simulink model "new_model_like_me"  (R2023a)
settings: Solver=FixedStepDiscrete  StartTime=0.0  StopTime=5  FixedStep=Ts  RelTol=1e-3  EnableMultiTasking=on
PreLoadFcn:
  | parameters_for_model_inn;
StopFcn:
  | ee_addSimlogTimeStamp(bdroot)
values from neighbouring files (symbols this model uses):
  deg = 10    [parameters_for_model_inn.m]
  Jm = 0.001368    [parameters_for_model_inn.m]
  Kaw_omega = 1    [parameters_for_model_inn.m]
  Ki_id = 3    [parameters_for_model_inn.m]
  Ki_iq = 20    [parameters_for_model_inn.m]
  Ki_omega = 2.2    [parameters_for_model_inn.m]
  Kp_id = 0.01    [parameters_for_model_inn.m]
  Kp_iq = 1.8    [parameters_for_model_inn.m]
  Kp_omega = 0.6    [parameters_for_model_inn.m]
  Kp_pos = 0.8    [parameters_for_model_inn.m]
  Ld = 0.00595    [parameters_for_model_inn.m]
  LimA2down = -80    [parameters_for_model_inn.m]
  LimA2up = 64    [parameters_for_model_inn.m]
  Lq = 0.00595    [parameters_for_model_inn.m]
  p = 4    [parameters_for_model_inn.m]
  psim = 0.180694733685904    (= 0.180694733686)    [parameters_for_model_inn.m]
  Red = 34.68    [parameters_for_model_inn.m]
  Tid_start = Tiq_stop + 0.02    (= 0.1)    [parameters_for_model_inn.m]
  Tid_stop = Tid_start + 0.04    (= 0.14)    [parameters_for_model_inn.m]
  Tiq_start = 0.02    [parameters_for_model_inn.m]
  Tiq_stop = Tiq_start + 0.06    (= 0.08)    [parameters_for_model_inn.m]
  Tomega_start = Tid_stop + 0.02    (= 0.16)    [parameters_for_model_inn.m]
  Tomega_stop = Tomega_start + 0.06    (= 0.22)    [parameters_for_model_inn.m]
  Tpos_start = Tomega_stop + 0.02    (= 0.24)    [parameters_for_model_inn.m]
  Tpos_stop = Tpos_start + 0.06    (= 0.3)    [parameters_for_model_inn.m]
  Ts = 5e-5    (= 5e-05)    [parameters_for_model_inn.m]
  Tsi = Ts * 20    (= 0.001)    [parameters_for_model_inn.m]
  Tso = Ts * 200    (= 0.01)    [parameters_for_model_inn.m]
  V1 = 250    [parameters_for_model_inn.m]
  Vnom = 300    [parameters_for_model_inn.m]
  Wmax = 7000    [parameters_for_model_inn.m]
  Wnom = 1800    [parameters_for_model_inn.m]
undefined symbols (not defined in the file or in its folder): DiscIntNeverNeededParam, Kd_pos, Ki_pos, Kn_pos, Tpos, X, Y, Z
libraries: nesl_utility x18, fl_lib x10, sm_lib x8, slctrlblks x6, ee_lib x5, eeTransforms x3, dspfdesign x3, eePmsmCurrentController x2, simulink x2, slpidlib x2, robotmaniplib x2, batteryecm_lib x1
(part 2 of 2)

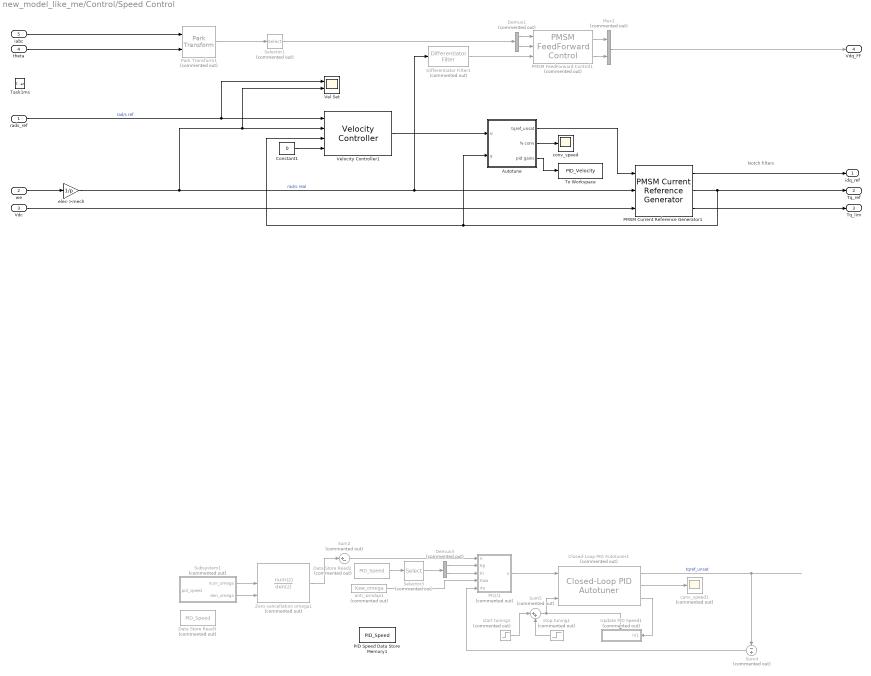
== system new_model_like_me/Control/Speed Control ==
  note: Notch filters
  rads_ref : Inport
  we : Inport  Port=2
  Vdc : Inport  Port=3
  theta : Inport  Port=4
  iabc : Inport  Port=5
  Task1ms : TriggerPort  TriggerType=function-call  VariantControl=Variant  PortDimensions=1
  Autotune : Subsystem
  Closed-Loop PID Autotuner1 : slctrlblks/Closed-Loop PID Autotuner  Commented=on  PIDType=PI  PIDForm=Parallel  TimeDomain=discrete-time  DiscreteTs=-1  TuningTs=0.2  UseTuningTs=off  IntegratorFormula=Forward Euler  FilterFormula=Forward Euler  ContinuousTs=0.02  Bandwidth=Wnom*(2*pi/60)  UseExternalWC=off  TargetPM=60  UseExternalPM=off  UseExternalAchievedPM=off  ExperimentMode=Superposition  PlantType=Stable  PlantSign=Positive  AmpSine=0.3  UseExternalAmpSine=off  UseExternalFRD=off  UseExternalU0=off  UseCompanion=off  NotDeployTuningModule=off  UsePLCCoder=off  OutputMode=control action + perturbation  BlockDataType=double  UseConnectedPID=on  blockpath=[]  tunedP=0  tunedI=0  tunedD=0  tunedN=100  tunedPM=0  EstimationWindowSize=3  UseExternalTuningParams=off  SingleMultiRateVariant=SingleSamplingRate  NumEstimationPeriods=4  NumSettlingPeriods=2  ExperimentModeVariant=VariantSuperimposed  OutputChoice=VariantCandD
  Constant1 : Constant  Value=0  SampleTime=-1
  Data Store Read2 : DataStoreRead  Commented=on  DataStoreName=PID_Speed  IndexOptions=Index vector (dialog)  Indices=1  OutputSizes=1
  Data Store Read3 : DataStoreRead  Commented=on  DataStoreName=PID_Speed  IndexOptions=Index vector (dialog)  Indices=1  OutputSizes=1
  Demux1 : Demux  Commented=on  Outputs=2
  Demux3 : Demux  Commented=on  Outputs=2
  Differentiator Filter1 : dspfdesign/Differentiator Filter  Commented=on  DesignForMinimumOrder=on  FilterOrder=31  PassbandRipple=0.1  ScaleCoefficients=off  SimulateUsing=Interpreted execution  roundingMode=Floor  coeffsDataTypeStr=fixdt(1,16)
  Mux1 : Mux  Commented=on  Inputs=2
  PI(z)1 : Subsystem  Commented=on
  PID Speed Data Store Memory1 : DataStoreMemory  DataStoreName=PID_Speed  InitialValue=[Kp_omega Ki_omega 0 Kaw_omega]  ShowAdditionalParam=off
  PMSM Current Reference Generator1 : eePmsmCurrentReferenceGen/PMSM Current Reference Generator  Vnom=Vnom  Pmax=Pmax  Tmax=Tmax  Ts=-1  RefType=Zero d-axis control  rpmVec=RPM_VECT  TqVec=TQ_VECT  VdcVec=VDC_VECT  PWMMode=SVM: space vector modulation  ModFactor=1  idMatrix=ID_MAP  iqMatrix=IQ_MAP  p=p  psim=psim  Ld=Ld  Lq=Lq  Rs=Rs  RefExpEnable=1
  PMSM FeedForward Control1 : mcbpmsmnonlinearlib/PMSM FeedForward Control  Commented=on  polePairs=p  nonLinearityChoice=Linear model with lumped parameters  Ld=Ld  Lq=Lq  FluxPM=psim  idVec=[-40, -20, 0, 20]  iqVec=[-40, -20, 0, 20, 40]  LdTable=0.2e-3 * ones(4, 5)  LqTable=0.2e-3 * ones(4, 5)  FluxPMTable=6.4e-3 * ones(4, 5)  FluxDTable=[-1.6,-1.6,-1.6,-1.6,-1.6;2.4,2.4,2.4,2.4,2.4;6.4,6.4,6.4,6.4,6.4;10.4,10.4,10.4,10.4,10.4]*1e-3  FluxQTable=[-8,-4,0,4,8;-8,-4,0,4,8;-8,-4,0,4,8;-8,-4,0,4,8]*1e-3  Vsat_input_select=Specify via dialog  v_sat=Vnom/sqrt(3)  Units=Per-Unit (PU)  V_base=Vnom/sqrt(3)  I_base=Imax  N_base=Wmax  scaledTables=on
      settings: LibrarySourceBlock=mcblib/Controls/Control Reference/PMSM FeedForward Control
  Park Transform1 : eeTransforms/Park Transform  Commented=on  AxisAlignment=Q-axis  PowerInvariant=off
      settings: LibrarySourceBlock=|
      | ee_sl_lib/Mathematical
      | Transforms/Park Transform
  Selector1 : Selector  Commented=on  InputPortWidth=3  IndexOptions=Index vector (dialog)  Indices=[1 2]  OutputSizes=1
  Selector3 : Selector  Commented=on  InputPortWidth=4  IndexOptions=Index vector (dialog)  Indices=[1 2]  OutputSizes=1
  Subsystem1 : Subsystem  Commented=on
  Sum2 : Sum  Commented=on  Inputs=|+-
  Sum4 : Sum  Commented=on  Inputs=-+
  Sum5 : Sum  Commented=on  Inputs=|++
  To Workspace : ToWorkspace  VariableName=PID_Velocity  SampleTime=-1
  Update PID Speed1 : Subsystem  Commented=on
  Vel Set : Scope  NumInputPorts=2
  Velocity Controller1 : eeVelocityController/Velocity Controller  CtrlType=P-PI control  Kp_w=Kp_omega  Ki_w=Ki_omega  Kv_w=P_omega  Kaw_w=Kaw_omega  Ts=-1  Tsd=Tso  ActZC=on
  Zero-cancellation omega1 : DiscreteTransferFcn  Commented=on  NumeratorSource=Input port  Numerator=(Tso*Ki_omega)/Kp_omega  DenominatorSource=Input port  Denominator=[1, ((Tso - Kp_omega/Ki_omega)/(Kp_omega/Ki_omega))]  a0EqualsOne=on
      settings: InputPortMap=u0,p1,p3
  anti_windup1 : Constant  Commented=on  Value=Kaw_omega
  conv_speed : Scope
  conv_speed1 : Scope  Commented=on
  elec->mech : Gain  Gain=1/p
  start tuning1 : Step  Commented=on  Time=Tomega_start
  stop tuning1 : Step  Commented=on  Time=Tomega_stop  After=-1
  idq_ref : Outport  VectorParamsAs1DForOutWhenUnconnected=off
  Tq_ref : Outport  Port=2  VectorParamsAs1DForOutWhenUnconnected=off
  Tq_lim : Outport  Port=3  VectorParamsAs1DForOutWhenUnconnected=off
  Vdq_FF : Outport  Port=4
  wires:
  we/1 -> elec->mech/1
  PMSM Current Reference Generator1/1 -> idq_ref/1
  PMSM Current Reference Generator1/3 -> Tq_lim/1
  Demux1/1 -> PMSM FeedForward Control1/1
  iabc/1 -> Park Transform1/1
  Velocity Controller1/1 -> Autotune/1(u)
  Park Transform1/1 -> Selector1/1
  Constant1/1 -> Velocity Controller1/4
  Selector1/1 -> Demux1/1
  rads_ref/1 -> Vel Set/1, Velocity Controller1/1  "rad/s ref"
  Differentiator Filter1/1 -> PMSM FeedForward Control1/3
  theta/1 -> Park Transform1/2
  Demux1/2 -> PMSM FeedForward Control1/2
  elec->mech/1 -> Vel Set/2, Velocity Controller1/2, Differentiator Filter1/1, PMSM Current Reference Generator1/2  "rad/s real"
  Vdc/1 -> PMSM Current Reference Generator1/3
  PMSM Current Reference Generator1/2 -> Autotune/2(y), Velocity Controller1/3, Tq_ref/1
  PMSM FeedForward Control1/2 -> Mux1/2
  PMSM FeedForward Control1/1 -> Mux1/1
  Subsystem1/1(num_omega) -> Zero-cancellation omega1/2
  Sum5/1 -> Closed-Loop PID Autotuner1/3, Update PID Speed1/Trigger
  start tuning1/1 -> Sum5/1
  Closed-Loop PID Autotuner1/2 -> conv_speed1/1
  ? -> Zero-cancellation omega1/1
  Selector3/1 -> Demux3/1
  Data Store Read2/1 -> Selector3/1
  PI(z)1/1(u) -> Closed-Loop PID Autotuner1/1
  ? -> Sum2/2, Closed-Loop PID Autotuner1/2  "wMech"
  Sum2/1 -> PI(z)1/1(e)
  anti_windup1/1 -> PI(z)1/4(Kaw)
  Closed-Loop PID Autotuner1/1 -> Sum4/1  "tqref_unsat"
  Sum4/1 -> PI(z)1/5(du)
  Demux3/2 -> PI(z)1/3(Ki)
  ? -> Sum4/2
  Zero-cancellation omega1/1 -> Sum2/1
  Closed-Loop PID Autotuner1/3 -> Update PID Speed1/1(In1)
  stop tuning1/1 -> Sum5/2
  Demux3/1 -> PI(z)1/2(Kp)
  Subsystem1/2(den_omega) -> Zero-cancellation omega1/3
  Mux1/1 -> Vdq_FF/1
  Autotune/1(tqref_unsat) -> PMSM Current Reference Generator1/1
  Autotune/2(% conv) -> conv_speed/1
  Autotune/3(pid gains) -> To Workspace/1

== system new_model_like_me/Load with Link/Link1 ==
  Link1 : sm_lib/Body Elements/File Solid  ExtGeomFileName=C:\Users\sk1nn\Documents\GitHub\MatLab\RX-50_simulink\STP_3d_model\Joint 1.stp  UnitType=FromFile  ExtGeomFileUnits=m  StepReaderType=HEX  ExportConvexHullGeometry=off  InertiaType=CalculateFromGeometry  Mass=147871.26  MassUnits=g  CenterOfMass=[0.11048, 0.013358, 0.110692]  CenterOfMassUnits=m  MomentsOfInertia=[1 1 1]  MomentsOfInertiaUnits=kg*m^2  ProductsOfInertia=[0 0 0]  ProductsOfInertiaUnits=kg*m^2  BasedOnType=Mass  Density=1000  DensityUnits=kg/m^3  DoExposeReferenceFrame=off  SerializedFrames=<Frames><Frame><Id>Frame1</Id><Value><Name>F1</Name><Origin><Source>GeometricFeature</Source><FeatureName>circular curve 3021</FeatureName></Origin><PrimaryAxis><DefinedDirection>+Z</DefinedDirection><Source>ReferenceFrame</Source><SourceDirection>+Z</SourceDirection><FeatureName></FeatureName></PrimaryAxis><SecondaryAxis><DefinedDirection>+X</DefinedDirection><Source>ReferenceFrame</Source><SourceDirection>+X</SourceDirection><FeatureName></FeatureName></SecondaryAxis></Value></Frame></Frames>  GraphicType=FromGeometry  MarkerShape=Sphere  MarkerSize=10  GraphicVisPropType=SimpleVisualProperties  GraphicDiffuseColor=[0.5 0.5 0.5]  GraphicSpecularColor=[0.5 0.5 0.5 1.0]  GraphicAmbientColor=[0.15 0.15 0.15 1.0]  GraphicEmissiveColor=[0.0 0.0 0.0 1.0]  GraphicShininess=75  GraphicOpacity=1.0
  j1 to link 1 : sm_lib/Frames and Transforms/Rigid Transform  TranslationMethod=Cartesian  TranslationStandardOffset=0  TranslationStandardOffsetUnits=mm  TranslationStandardAxis=+Z  TranslationCartesianOffset=[0 0 0]  TranslationCartesianOffsetUnits=mm  TranslationROffset=0  TranslationROffsetUnits=m  TranslationZOffset=0  TranslationZOffsetUnits=m  TranslationThetaOffset=0  TranslationThetaOffsetUnits=deg  RotationMethod=None  RotationAngleUnits=deg  RotationStandardAxis=+Z  RotationAngle=0.0  RotationArbitraryAxis=[0 0 1]  FollAlignAxisA=+X  BaseAlignAxisA=+Y  FollAlignAxisB=+Y  BaseAlignAxisB=+Z  RotationSequenceAxes=FollowerAxes  RotationSequence=XYX  RotationSequenceAngles=[0 0 0]  RotationSequenceAnglesUnits=deg  RotationMatrix=[1 0 0; 0 1 0; 0 0 1]  Quaternion=[1 0 0 0]
  link1 to j2 : sm_lib/Frames and Transforms/Rigid Transform  TranslationMethod=Cartesian  TranslationStandardOffset=0  TranslationStandardOffsetUnits=mm  TranslationStandardAxis=+X  TranslationCartesianOffset=[265 -153 240]  TranslationCartesianOffsetUnits=mm  TranslationROffset=0  TranslationROffsetUnits=m  TranslationZOffset=0  TranslationZOffsetUnits=m  TranslationThetaOffset=0  TranslationThetaOffsetUnits=deg  RotationMethod=StandardAxis  RotationAngleUnits=deg  RotationStandardAxis=+X  RotationAngle=90  RotationArbitraryAxis=[0 0 1]  FollAlignAxisA=+X  BaseAlignAxisA=+Y  FollAlignAxisB=+Y  BaseAlignAxisB=+Z  RotationSequenceAxes=FollowerAxes  RotationSequence=XYX  RotationSequenceAngles=[0 0 0]  RotationSequenceAnglesUnits=deg  RotationMatrix=[1 0 0; 0 1 0; 0 0 1]  Quaternion=[1 0 0 0]
  J2 : PMIOPort  Side=Right
  J1 : PMIOPort  Port=2  Side=Left
  connections:
  j1 to link 1/RConn1 -- Link1/LConn1 -- link1 to j2/LConn1
  link1 to j2/RConn1 -- J2/RConn1
  j1 to link 1/LConn1 -- J1/RConn1

== system new_model_like_me/Load with Link/Link2_1 ==
  Link2_1 : sm_lib/Body Elements/File Solid  ExtGeomFileName=C:\Users\sk1nn\Documents\GitHub\MatLab\RX-50_simulink\STP_3d_model\Joint 2.stp  UnitType=FromFile  ExtGeomFileUnits=m  StepReaderType=HEX  ExportConvexHullGeometry=off  InertiaType=CalculateFromGeometry  Mass=27.33  MassUnits=kg  CenterOfMass=[0 0 0]  CenterOfMassUnits=m  MomentsOfInertia=[1 1 1]  MomentsOfInertiaUnits=kg*m^2  ProductsOfInertia=[0 0 0]  ProductsOfInertiaUnits=kg*m^2  BasedOnType=Mass  Density=1000  DensityUnits=kg/m^3  DoExposeReferenceFrame=off  SerializedFrames=<Frames><Frame><Id>Frame1</Id><Value><Name>F1</Name><Origin><Source>CenterOfMassFrame</Source><FeatureName></FeatureName></Origin><PrimaryAxis><DefinedDirection>+Z</DefinedDirection><Source>ReferenceFrame</Source><SourceDirection>+Z</SourceDirection><FeatureName></FeatureName></PrimaryAxis><SecondaryAxis><DefinedDirection>+X</DefinedDirection><Source>ReferenceFrame</Source><SourceDirection>+X</SourceDirection><FeatureName></FeatureName></SecondaryAxis></Value></Frame></Frames>  GraphicType=FromGeometry  MarkerShape=Sphere  MarkerSize=10  GraphicVisPropType=SimpleVisualProperties  GraphicDiffuseColor=[0.5 0.5 0.5]  GraphicSpecularColor=[0.5 0.5 0.5 1.0]  GraphicAmbientColor=[0.15 0.15 0.15 1.0]  GraphicEmissiveColor=[0.0 0.0 0.0 1.0]  GraphicShininess=75  GraphicOpacity=1.0
  j2 to link 2_1 : sm_lib/Frames and Transforms/Rigid Transform  TranslationMethod=Cartesian  TranslationStandardOffset=0  TranslationStandardOffsetUnits=mm  TranslationStandardAxis=+Z  TranslationCartesianOffset=[0 320 20]  TranslationCartesianOffsetUnits=mm  TranslationROffset=0  TranslationROffsetUnits=m  TranslationZOffset=0  TranslationZOffsetUnits=m  TranslationThetaOffset=0  TranslationThetaOffsetUnits=deg  RotationMethod=StandardAxis  RotationAngleUnits=deg  RotationStandardAxis=+X  RotationAngle=-90  RotationArbitraryAxis=[0 0 1]  FollAlignAxisA=+X  BaseAlignAxisA=+Y  FollAlignAxisB=+Y  BaseAlignAxisB=+Z  RotationSequenceAxes=FollowerAxes  RotationSequence=XYX  RotationSequenceAngles=[0 0 0]  RotationSequenceAnglesUnits=deg  RotationMatrix=[1 0 0; 0 1 0; 0 0 1]  Quaternion=[1 0 0 0]
  J2 : PMIOPort  Side=Left
  connections:
  Link2_1/LConn1 -- j2 to link 2_1/RConn1
  j2 to link 2_1/LConn1 -- J2/RConn1

== system new_model_like_me/Load with Link/Reductor ==
  rad : Inport
  Gain : Gain  Gain=1/Red
  rad_red : Outport
  wires:
  Gain/1 -> rad_red/1
  rad/1 -> Gain/1

== system new_model_like_me/Load with Link/Reductor_check ==
  trq : Inport
  Gain : Gain  Gain=1/Red
  trq_red : Outport
  wires:
  Gain/1 -> trq_red/1
  trq/1 -> Gain/1

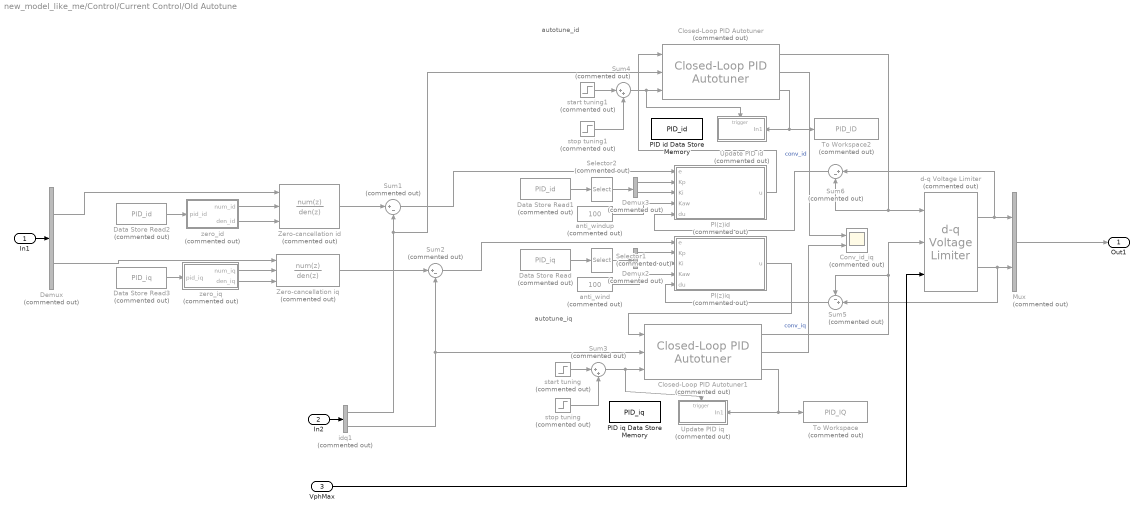
== system new_model_like_me/Control/Current Control/Old Autotune ==
  note: autotune_iq
  note: autotune_id
  In1 : Inport
  In2 : Inport  Port=2
  VphMax : Inport  Port=3
  Closed-Loop PID Autotuner : slctrlblks/Closed-Loop PID Autotuner  Commented=on  PIDType=PI  PIDForm=Parallel  TimeDomain=discrete-time  DiscreteTs=-1  TuningTs=0.2  UseTuningTs=off  IntegratorFormula=Forward Euler  FilterFormula=Forward Euler  ContinuousTs=0.02  Bandwidth=Imax  UseExternalWC=off  TargetPM=60  UseExternalPM=off  UseExternalAchievedPM=off  ExperimentMode=Superposition  PlantType=Stable  PlantSign=Positive  AmpSine=0.03  UseExternalAmpSine=off  UseExternalFRD=off  UseExternalU0=off  UseCompanion=off  NotDeployTuningModule=off  UsePLCCoder=off  OutputMode=control action + perturbation  BlockDataType=double  UseConnectedPID=on  blockpath=[]  tunedP=0  tunedI=0  tunedD=0  tunedN=100  tunedPM=0  EstimationWindowSize=3  UseExternalTuningParams=off  SingleMultiRateVariant=SingleSamplingRate  NumEstimationPeriods=4  NumSettlingPeriods=2  ExperimentModeVariant=VariantSuperimposed  OutputChoice=VariantCandD
  Closed-Loop PID Autotuner1 : slctrlblks/Closed-Loop PID Autotuner  Commented=on  PIDType=PI  PIDForm=Parallel  TimeDomain=discrete-time  DiscreteTs=-1  TuningTs=0.2  UseTuningTs=off  IntegratorFormula=Forward Euler  FilterFormula=Forward Euler  ContinuousTs=0.02  Bandwidth=Imax  UseExternalWC=off  TargetPM=60  UseExternalPM=off  UseExternalAchievedPM=off  ExperimentMode=Superposition  PlantType=Stable  PlantSign=Positive  AmpSine=0.03  UseExternalAmpSine=off  UseExternalFRD=off  UseExternalU0=off  UseCompanion=off  NotDeployTuningModule=off  UsePLCCoder=off  OutputMode=control action + perturbation  BlockDataType=double  UseConnectedPID=on  blockpath=[]  tunedP=0  tunedI=0  tunedD=0  tunedN=100  tunedPM=0  EstimationWindowSize=3  UseExternalTuningParams=off  SingleMultiRateVariant=SingleSamplingRate  NumEstimationPeriods=4  NumSettlingPeriods=2  ExperimentModeVariant=VariantSuperimposed  OutputChoice=VariantCandD
  Conv_id_iq : Scope  Commented=on  NumInputPorts=2
  Data Store Read : DataStoreRead  Commented=on  DataStoreName=PID_iq  IndexOptions=Index vector (dialog)  Indices=1  OutputSizes=1
  Data Store Read1 : DataStoreRead  Commented=on  DataStoreName=PID_id  IndexOptions=Index vector (dialog)  Indices=1  OutputSizes=1
  Data Store Read2 : DataStoreRead  Commented=on  DataStoreName=PID_id  IndexOptions=Index vector (dialog)  Indices=1  OutputSizes=1
  Data Store Read3 : DataStoreRead  Commented=on  DataStoreName=PID_iq  IndexOptions=Index vector (dialog)  Indices=1  OutputSizes=1
  Demux : Demux  Commented=on  Outputs=2
  Demux2 : Demux  Commented=on  Outputs=2
  Demux3 : Demux  Commented=on  Outputs=2
  Mux : Mux  Commented=on  Inputs=2
  PI(z)id : Subsystem  Commented=on
  PI(z)iq : Subsystem  Commented=on
  PID id Data Store Memory : DataStoreMemory  DataStoreName=PID_id  InitialValue=[Kp_id Ki_id 0 100]  ShowAdditionalParam=off
  PID iq Data Store Memory : DataStoreMemory  DataStoreName=PID_iq  InitialValue=[Kp_iq Ki_iq 0 100]  ShowAdditionalParam=off
  Selector1 : Selector  Commented=on  InputPortWidth=4  IndexOptions=Index vector (dialog)  Indices=[1 2]  OutputSizes=1
  Selector2 : Selector  Commented=on  InputPortWidth=4  IndexOptions=Index vector (dialog)  Indices=[1 2]  OutputSizes=1
  Sum1 : Sum  Commented=on  Inputs=|+-
  Sum2 : Sum  Commented=on  Inputs=|+-
  Sum3 : Sum  Commented=on  Inputs=|++
  Sum4 : Sum  Commented=on  Inputs=|++
  Sum5 : Sum  Commented=on  Inputs=-+|
  Sum6 : Sum  Commented=on  Inputs=|+-
  To Workspace : ToWorkspace  Commented=on  VariableName=PID_IQ  SampleTime=-1
      settings: Save2DSignal=2-D array (concatenate along first dimension)
  To Workspace2 : ToWorkspace  Commented=on  VariableName=PID_ID  SampleTime=-1
      settings: Save2DSignal=2-D array (concatenate along first dimension)
  Update PID id : Subsystem  Commented=on
  Update PID iq : Subsystem  Commented=on
  Zero-cancellation id : DiscreteTransferFcn  Commented=on  NumeratorSource=Input port  Numerator=(Tsi*Ki_id)/(Kp_id)  DenominatorSource=Input port  Denominator=[1, ((Tsi-Kp_id/Ki_id)/(Kp_id/Ki_id))]  a0EqualsOne=on
      settings: InputPortMap=u0,p1,p3
  Zero-cancellation iq : DiscreteTransferFcn  Commented=on  NumeratorSource=Input port  Numerator=(Tsi*Ki_iq)/(Kp_iq)  DenominatorSource=Input port  Denominator=[1, ((Tsi-Kp_iq/Ki_iq)/(Kp_iq/Ki_iq))]  a0EqualsOne=on
      settings: InputPortMap=u0,p1,p3
  anti_wind : Constant  Commented=on  Value=100
  anti_windup : Constant  Commented=on  Value=100
  d-q Voltage Limiter : eeDqVoltageLimiter/d-q Voltage Limiter  Commented=on  AxisPrio=Q-axis  Ts=-1
      settings: LibrarySourceBlock=|
      | eePmsmCurrentController/PMSM Current Controller
      | with Pre-Control/d-q Voltage Limiter
  idq1 : Demux  Commented=on  Outputs=2
  start tuning : Step  Commented=on  Time=Tiq_start
  start tuning1 : Step  Commented=on  Time=Tid_start
  stop tuning : Step  Commented=on  Time=Tiq_stop  After=-1
  stop tuning1 : Step  Commented=on  Time=Tid_stop  After=-1
  zero_id : Subsystem  Commented=on
  zero_iq : Subsystem  Commented=on
  Out1 : Outport
  wires:
  In1/1 -> Demux/1
  In2/1 -> idq1/1
  stop tuning/1 -> Sum3/2
  Mux/1 -> Out1/1
  Closed-Loop PID Autotuner/3 -> To Workspace2/1, Update PID id/1(In1)
  idq1/1 -> Closed-Loop PID Autotuner/2, Sum1/2
  anti_wind/1 -> PI(z)iq/4(Kaw)
  Sum4/1 -> Update PID id/Trigger, Closed-Loop PID Autotuner/3
  Sum6/1 -> PI(z)id/5(du)
  Closed-Loop PID Autotuner1/2 -> Conv_id_iq/2  "conv_iq"
  d-q Voltage Limiter/2 -> Sum5/2, Mux/2
  Data Store Read/1 -> Selector1/1
  zero_id/1(num_id) -> Zero-cancellation id/2
  Demux2/2 -> PI(z)iq/3(Ki)
  Closed-Loop PID Autotuner1/1 -> d-q Voltage Limiter/2, Sum5/1
  Closed-Loop PID Autotuner/1 -> d-q Voltage Limiter/1, Sum6/2
  Selector1/1 -> Demux2/1
  Closed-Loop PID Autotuner/2 -> Conv_id_iq/1  "conv_id"
  start tuning/1 -> Sum3/1
  Sum5/1 -> PI(z)iq/5(du)
  Data Store Read1/1 -> Selector2/1
  Sum1/1 -> PI(z)id/1(e)
  Closed-Loop PID Autotuner1/3 -> To Workspace/1, Update PID iq/1(In1)
  stop tuning1/1 -> Sum4/2
  Zero-cancellation id/1 -> Sum1/1
  zero_id/2(den_id) -> Zero-cancellation id/3
  Sum3/1 -> Update PID iq/Trigger, Closed-Loop PID Autotuner1/3
  idq1/2 -> Closed-Loop PID Autotuner1/2, Sum2/2
  Demux2/1 -> PI(z)iq/2(Kp)
  start tuning1/1 -> Sum4/1
  d-q Voltage Limiter/1 -> Sum6/1, Mux/1
  Zero-cancellation iq/1 -> Sum2/1
  Demux/1 -> Zero-cancellation id/1
  zero_iq/1(num_iq) -> Zero-cancellation iq/2
  PI(z)id/1(u) -> Closed-Loop PID Autotuner/1
  Demux3/1 -> PI(z)id/2(Kp)
  Sum2/1 -> PI(z)iq/1(e)
  PI(z)iq/1(u) -> Closed-Loop PID Autotuner1/1
  Demux3/2 -> PI(z)id/3(Ki)
  Selector2/1 -> Demux3/1
  Data Store Read2/1 -> zero_id/1(pid_id)
  anti_windup/1 -> PI(z)id/4(Kaw)
  Data Store Read3/1 -> zero_iq/1(pid_iq)
  Demux/2 -> Zero-cancellation iq/1
  zero_iq/2(den_iq) -> Zero-cancellation iq/3
  VphMax/1 -> d-q Voltage Limiter/3

== system new_model_like_me/Control/Measurements/Vdc Filter ==
  In : Inport
  Discrete Transfer Fcn : DiscreteTransferFcn  Numerator=num  Denominator=den
  Out : Outport  VectorParamsAs1DForOutWhenUnconnected=off
  wires:
  Discrete Transfer Fcn/1 -> Out/1
  In/1 -> Discrete Transfer Fcn/1

== system new_model_like_me/Control/Position Control/Autotune ==
  rad_aft_pid : Inport
  real_rad : Inport  Port=2
  start/stop : Inport  Port=3
  Closed-Loop PID Autotuner : slctrlblks/Closed-Loop PID Autotuner  PIDType=PID  PIDForm=Parallel  TimeDomain=discrete-time  DiscreteTs=-1  TuningTs=0.2  UseTuningTs=off  IntegratorFormula=Forward Euler  FilterFormula=Forward Euler  ContinuousTs=0.02  Bandwidth=31  UseExternalWC=off  TargetPM=60  UseExternalPM=off  UseExternalAchievedPM=off  ExperimentMode=Superposition  PlantType=Stable  PlantSign=Positive  AmpSine=0.3  UseExternalAmpSine=off  UseExternalFRD=off  UseExternalU0=off  UseCompanion=off  NotDeployTuningModule=off  UsePLCCoder=off  OutputMode=control action + perturbation  BlockDataType=double  UseConnectedPID=on  blockpath=[]  tunedP=0  tunedI=0  tunedD=0  tunedN=100  tunedPM=0  EstimationWindowSize=3  UseExternalTuningParams=off  SingleMultiRateVariant=SingleSamplingRate  NumEstimationPeriods=4  NumSettlingPeriods=2  ExperimentModeVariant=VariantSuperimposed  OutputChoice=VariantCandD
  conv_pos : Scope
  out : Outport
  pid gains : Outport  Port=2
  wires:
  real_rad/1 -> Closed-Loop PID Autotuner/2
  Closed-Loop PID Autotuner/2 -> conv_pos/1
  Closed-Loop PID Autotuner/1 -> out/1
  Closed-Loop PID Autotuner/3 -> pid gains/1
  rad_aft_pid/1 -> Closed-Loop PID Autotuner/1
  start/stop/1 -> Closed-Loop PID Autotuner/3

== system new_model_like_me/Control/Position Control/Autotune1 ==
  rad_aft_pid : Inport
  real_rad : Inport  Port=2
  Closed-Loop PID Autotuner : slctrlblks/Closed-Loop PID Autotuner  PIDType=P  PIDForm=Parallel  TimeDomain=discrete-time  DiscreteTs=-1  TuningTs=0.2  UseTuningTs=off  IntegratorFormula=Forward Euler  FilterFormula=Forward Euler  ContinuousTs=0.02  Bandwidth=(LimA2up-LimA2down)*pi/180  UseExternalWC=off  TargetPM=60  UseExternalPM=off  UseExternalAchievedPM=off  ExperimentMode=Superposition  PlantType=Stable  PlantSign=Positive  AmpSine=0.3  UseExternalAmpSine=off  UseExternalFRD=off  UseExternalU0=off  UseCompanion=off  NotDeployTuningModule=off  UsePLCCoder=off  OutputMode=control action + perturbation  BlockDataType=double  UseConnectedPID=on  blockpath=[]  tunedP=0  tunedI=0  tunedD=0  tunedN=100  tunedPM=0  EstimationWindowSize=3  UseExternalTuningParams=off  SingleMultiRateVariant=SingleSamplingRate  NumEstimationPeriods=4  NumSettlingPeriods=2  ExperimentModeVariant=VariantSuperimposed  OutputChoice=VariantCandD
  Sum2 : Sum  Inputs=|++
  conv_pos : Scope
  start tuning : Step  Time=Tpos_start
  stop tuning : Step  Time=Tpos_stop  After=-1
  out : Outport
  pid gains : Outport  Port=2
  wires:
  real_rad/1 -> Closed-Loop PID Autotuner/2
  Closed-Loop PID Autotuner/2 -> conv_pos/1
  Closed-Loop PID Autotuner/1 -> out/1
  Closed-Loop PID Autotuner/3 -> pid gains/1
  rad_aft_pid/1 -> Closed-Loop PID Autotuner/1
  Sum2/1 -> Closed-Loop PID Autotuner/3
  start tuning/1 -> Sum2/1
  stop tuning/1 -> Sum2/2

== system new_model_like_me/Control/Position Control/Update PID Pos ==
  In1 : Inport
  Trigger : TriggerPort  TriggerType=falling  VariantControl=Variant  PortDimensions=1
  Bus Selector : BusSelector  OutputSignals=P,I,D,N
  Mux : Mux
  Write PID Gains : DataStoreWrite  DataStoreName=PID_Pos  IndexOptions=Index vector (dialog)  Indices=1  OutputSizes=1
  wires:
  Mux/1 -> Write PID Gains/1
  Bus Selector/2 -> Mux/2  "<I>"
  Bus Selector/1 -> Mux/1  "<P>"
  In1/1 -> Bus Selector/1
  Bus Selector/3 -> Mux/3  "<D>"
  Bus Selector/4 -> Mux/4  "<N>"

== system new_model_like_me/Control/Speed Control/Autotune ==
  u : Inport
  y : Inport  Port=2
  Closed-Loop PID Autotuner2 : slctrlblks/Closed-Loop PID Autotuner  PIDType=PI  PIDForm=Parallel  TimeDomain=discrete-time  DiscreteTs=-1  TuningTs=0.2  UseTuningTs=off  IntegratorFormula=Forward Euler  FilterFormula=Forward Euler  ContinuousTs=0.02  Bandwidth=Wnom*(2*pi/60)  UseExternalWC=off  TargetPM=60  UseExternalPM=off  UseExternalAchievedPM=off  ExperimentMode=Superposition  PlantType=Stable  PlantSign=Positive  AmpSine=0.4  UseExternalAmpSine=off  UseExternalFRD=off  UseExternalU0=off  UseCompanion=off  NotDeployTuningModule=off  UsePLCCoder=off  OutputMode=control action + perturbation  BlockDataType=double  UseConnectedPID=on  blockpath=[]  tunedP=0  tunedI=0  tunedD=0  tunedN=100  tunedPM=0  EstimationWindowSize=3  UseExternalTuningParams=off  SingleMultiRateVariant=SingleSamplingRate  NumEstimationPeriods=4  NumSettlingPeriods=2  ExperimentModeVariant=VariantSuperimposed  OutputChoice=VariantCandD
  Sum1 : Sum  Inputs=|++
  start tuning2 : Step  Time=Tomega_start
  stop tuning2 : Step  Time=Tomega_stop  After=-1
  tqref_unsat : Outport
  % conv : Outport  Port=2
  pid gains : Outport  Port=3
  wires:
  u/1 -> Closed-Loop PID Autotuner2/1
  Closed-Loop PID Autotuner2/2 -> % conv/1
  Sum1/1 -> Closed-Loop PID Autotuner2/3
  Closed-Loop PID Autotuner2/3 -> pid gains/1
  stop tuning2/1 -> Sum1/2
  y/1 -> Closed-Loop PID Autotuner2/2
  start tuning2/1 -> Sum1/1
  Closed-Loop PID Autotuner2/1 -> tqref_unsat/1  "tqref_unsat"

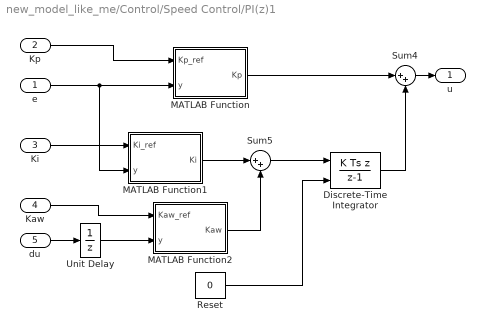
== system new_model_like_me/Control/Speed Control/PI(z)1 ==
  e : Inport
  Kp : Inport  Port=2
  Ki : Inport  Port=3
  Kaw : Inport  Port=4
  du : Inport  Port=5
  Discrete-Time Integrator : DiscreteIntegrator  IntegratorMethod=Integration: Backward Euler  ExternalReset=rising  SampleTime=-1  ICPrevOutput=DiscIntNeverNeededParam  ICPrevScaledInput=DiscIntNeverNeededParam
  MATLAB Function : MATLAB Function  TreatAsAtomicUnit=on
  MATLAB Function1 : MATLAB Function  TreatAsAtomicUnit=on
  MATLAB Function2 : MATLAB Function  TreatAsAtomicUnit=on
  Reset : Constant  Value=0
  Sum4 : Sum  Inputs=|++
  Sum5 : Sum  Inputs=|++
  Unit Delay : UnitDelay  SampleTime=-1  HasFrameUpgradeWarning=on
  u : Outport
  wires:
  MATLAB Function1/1(Ki) -> Sum5/1
  Sum4/1 -> u/1
  MATLAB Function2/1(Kaw) -> Sum5/2
  Unit Delay/1 -> MATLAB Function2/2(y)
  du/1 -> Unit Delay/1
  e/1 -> MATLAB Function1/2(y), MATLAB Function/2(y)
  MATLAB Function/1(Kp) -> Sum4/1
  Kp/1 -> MATLAB Function/1(Kp_ref)
  Ki/1 -> MATLAB Function1/1(Ki_ref)
  Kaw/1 -> MATLAB Function2/1(Kaw_ref)
  Sum5/1 -> Discrete-Time Integrator/1
  Discrete-Time Integrator/1 -> Sum4/2
  Reset/1 -> Discrete-Time Integrator/2

== system new_model_like_me/Control/Speed Control/Subsystem1 ==
  pid_speed : Inport
  Constant2 : Constant  Value=Tso
  Demux3 : Demux  Outputs=2
  Demux4 : Demux  Outputs=2
  MATLAB Function : MATLAB Function  TreatAsAtomicUnit=on
  MATLAB Function1 : MATLAB Function  TreatAsAtomicUnit=on
  Selector3 : Selector  InputPortWidth=4  IndexOptions=Index vector (dialog)  Indices=[1 2]  OutputSizes=1
  num_omega : Outport
  den_omega : Outport  Port=2
  wires:
  Demux3/2 -> MATLAB Function/2(Ki_omega)
  Selector3/1 -> Demux4/1, Demux3/1
  Demux4/2 -> MATLAB Function1/2(Ki_omega)
  Demux3/1 -> MATLAB Function/1(Kp_omega)
  Constant2/1 -> MATLAB Function/3(Tso), MATLAB Function1/3(Tso)
  Demux4/1 -> MATLAB Function1/1(Kp_omega)
  pid_speed/1 -> Selector3/1
  MATLAB Function/1(num_omega) -> num_omega/1
  MATLAB Function1/1(den_omega) -> den_omega/1

== system new_model_like_me/Control/Speed Control/Update PID Speed1 ==
  In1 : Inport
  Trigger : TriggerPort  TriggerType=falling  VariantControl=Variant  PortDimensions=1
  Bus Selector : BusSelector  OutputSignals=P,I,D,N
  Mux : Mux
  Write PID Gains : DataStoreWrite  DataStoreName=PID_Speed  IndexOptions=Index vector (dialog)  Indices=1  OutputSizes=1
  wires:
  Mux/1 -> Write PID Gains/1
  Bus Selector/2 -> Mux/2  "<I>"
  Bus Selector/1 -> Mux/1  "<P>"
  In1/1 -> Bus Selector/1
  Bus Selector/3 -> Mux/3  "<D>"
  Bus Selector/4 -> Mux/4  "<N>"

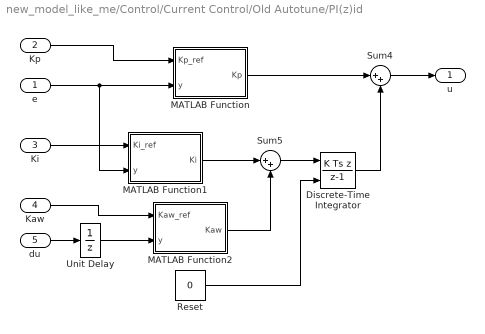
== system new_model_like_me/Control/Current Control/Old Autotune/PI(z)id ==
  e : Inport
  Kp : Inport  Port=2
  Ki : Inport  Port=3
  Kaw : Inport  Port=4
  du : Inport  Port=5
  Discrete-Time Integrator : DiscreteIntegrator  IntegratorMethod=Integration: Backward Euler  ExternalReset=rising  SampleTime=-1  ICPrevOutput=DiscIntNeverNeededParam  ICPrevScaledInput=DiscIntNeverNeededParam
  MATLAB Function : MATLAB Function  TreatAsAtomicUnit=on
  MATLAB Function1 : MATLAB Function  TreatAsAtomicUnit=on
  MATLAB Function2 : MATLAB Function  TreatAsAtomicUnit=on
  Reset : Constant  Value=0
  Sum4 : Sum  Inputs=|++
  Sum5 : Sum  Inputs=|++
  Unit Delay : UnitDelay  SampleTime=-1  HasFrameUpgradeWarning=on
  u : Outport
  wires:
  MATLAB Function1/1(Ki) -> Sum5/1
  Sum4/1 -> u/1
  Discrete-Time Integrator/1 -> Sum4/2
  MATLAB Function2/1(Kaw) -> Sum5/2
  Unit Delay/1 -> MATLAB Function2/2(y)
  du/1 -> Unit Delay/1
  e/1 -> MATLAB Function1/2(y), MATLAB Function/2(y)
  MATLAB Function/1(Kp) -> Sum4/1
  Kp/1 -> MATLAB Function/1(Kp_ref)
  Ki/1 -> MATLAB Function1/1(Ki_ref)
  Kaw/1 -> MATLAB Function2/1(Kaw_ref)
  Sum5/1 -> Discrete-Time Integrator/1
  Reset/1 -> Discrete-Time Integrator/2

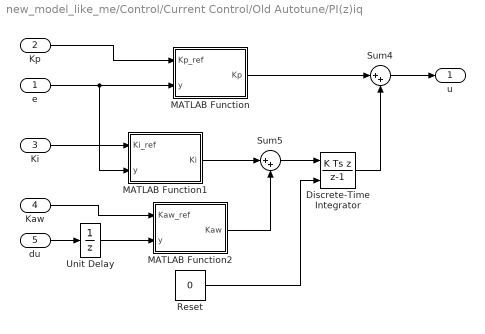
== system new_model_like_me/Control/Current Control/Old Autotune/PI(z)iq ==
  e : Inport
  Kp : Inport  Port=2
  Ki : Inport  Port=3
  Kaw : Inport  Port=4
  du : Inport  Port=5
  Discrete-Time Integrator : DiscreteIntegrator  IntegratorMethod=Integration: Backward Euler  ExternalReset=rising  SampleTime=-1  ICPrevOutput=DiscIntNeverNeededParam  ICPrevScaledInput=DiscIntNeverNeededParam
  MATLAB Function : MATLAB Function  TreatAsAtomicUnit=on
  MATLAB Function1 : MATLAB Function  TreatAsAtomicUnit=on
  MATLAB Function2 : MATLAB Function  TreatAsAtomicUnit=on
  Reset : Constant  Value=0
  Sum4 : Sum  Inputs=|++
  Sum5 : Sum  Inputs=|++
  Unit Delay : UnitDelay  SampleTime=-1  HasFrameUpgradeWarning=on
  u : Outport
  wires:
  MATLAB Function1/1(Ki) -> Sum5/1
  Sum4/1 -> u/1
  Discrete-Time Integrator/1 -> Sum4/2
  MATLAB Function2/1(Kaw) -> Sum5/2
  Unit Delay/1 -> MATLAB Function2/2(y)
  du/1 -> Unit Delay/1
  e/1 -> MATLAB Function1/2(y), MATLAB Function/2(y)
  MATLAB Function/1(Kp) -> Sum4/1
  Kp/1 -> MATLAB Function/1(Kp_ref)
  Ki/1 -> MATLAB Function1/1(Ki_ref)
  Kaw/1 -> MATLAB Function2/1(Kaw_ref)
  Sum5/1 -> Discrete-Time Integrator/1
  Reset/1 -> Discrete-Time Integrator/2

== system new_model_like_me/Control/Current Control/Old Autotune/Update PID id ==
  In1 : Inport
  Trigger : TriggerPort  TriggerType=falling  VariantControl=Variant  PortDimensions=1
  Bus Selector : BusSelector  OutputSignals=P,I,D,N
  Mux : Mux
  Write PID Gains : DataStoreWrite  DataStoreName=PID_id  IndexOptions=Index vector (dialog)  Indices=1  OutputSizes=1
  wires:
  Mux/1 -> Write PID Gains/1
  Bus Selector/2 -> Mux/2  "<I>"
  In1/1 -> Bus Selector/1
  Bus Selector/3 -> Mux/3  "<D>"
  Bus Selector/4 -> Mux/4  "<N>"
  Bus Selector/1 -> Mux/1  "<P>"

== system new_model_like_me/Control/Current Control/Old Autotune/Update PID iq ==
  In1 : Inport
  Trigger : TriggerPort  TriggerType=falling  VariantControl=Variant  PortDimensions=1
  Bus Selector : BusSelector  OutputSignals=P,I,D,N
  Mux : Mux
  Write PID Gains : DataStoreWrite  DataStoreName=PID_iq  IndexOptions=Index vector (dialog)  Indices=1  OutputSizes=1
  wires:
  Mux/1 -> Write PID Gains/1
  Bus Selector/2 -> Mux/2  "<I>"
  In1/1 -> Bus Selector/1
  Bus Selector/3 -> Mux/3  "<D>"
  Bus Selector/4 -> Mux/4  "<N>"
  Bus Selector/1 -> Mux/1  "<P>"

== system new_model_like_me/Control/Current Control/Old Autotune/zero_id ==
  pid_id : Inport
  Constant : Constant  Value=Tsi
  Demux4 : Demux  Outputs=2
  MATLAB Function : MATLAB Function  TreatAsAtomicUnit=on
  MATLAB Function3 : MATLAB Function  TreatAsAtomicUnit=on
  Selector3 : Selector  InputPortWidth=4  IndexOptions=Index vector (dialog)  Indices=[1 2]  OutputSizes=1
  num_id : Outport
  den_id : Outport  Port=2
  wires:
  Demux4/1 -> MATLAB Function3/1(Kp_id), MATLAB Function/1(Kp_id)
  Demux4/2 -> MATLAB Function/2(Ki_id), MATLAB Function3/2(Ki_id)
  Constant/1 -> MATLAB Function/3(Tsi), MATLAB Function3/3(Tsi)
  Selector3/1 -> Demux4/1
  MATLAB Function3/1(den_id) -> den_id/1
  MATLAB Function/1(num_id) -> num_id/1
  pid_id/1 -> Selector3/1

== system new_model_like_me/Control/Current Control/Old Autotune/zero_iq ==
  pid_iq : Inport
  Constant1 : Constant  Value=Tsi
  Demux5 : Demux  Outputs=2
  MATLAB Function1 : MATLAB Function  TreatAsAtomicUnit=on
  MATLAB Function2 : MATLAB Function  TreatAsAtomicUnit=on
  Selector4 : Selector  InputPortWidth=4  IndexOptions=Index vector (dialog)  Indices=[1 2]  OutputSizes=1
  num_iq : Outport
  den_iq : Outport  Port=2
  wires:
  Constant1/1 -> MATLAB Function1/3(Tsi), MATLAB Function2/3(Tsi)
  Demux5/2 -> MATLAB Function1/2(Ki_iq), MATLAB Function2/2(Ki_iq)
  Demux5/1 -> MATLAB Function1/1(Kp_iq), MATLAB Function2/1(Kp_iq)
  MATLAB Function1/1(num_iq) -> num_iq/1
  MATLAB Function2/1(den_iq) -> den_iq/1
  pid_iq/1 -> Selector4/1
  Selector4/1 -> Demux5/1

== matlab function new_model_like_me/Control/Current Control/Old Autotune/zero_iq/MATLAB Function2 ==
  data: Kp_iq input; den_iq output; Ki_iq input; Tsi input
function den_iq = fcn(Kp_iq, Ki_iq, Tsi)

den_iq = [1, ((Tsi-Kp_iq/Ki_iq)/(Kp_iq/Ki_iq))];

== matlab function new_model_like_me/Control/Current Control/Old Autotune/zero_id/MATLAB Function3 ==
  data: Kp_id input; den_id output; Ki_id input; Tsi input
function den_id = fcn(Kp_id, Ki_id, Tsi)

den_id = [1, ((Tsi-Kp_id/Ki_id)/(Kp_id/Ki_id))];

== matlab function new_model_like_me/Control/Current Control/Old Autotune/PI(z)id/MATLAB Function ==
  data: Kp_ref input; Kp output; y input
function Kp = fcn(Kp_ref, y)

Kp = Kp_ref*y;

== matlab function new_model_like_me/Control/Current Control/Old Autotune/PI(z)id/MATLAB Function1 ==
  data: Ki_ref input; Ki output; y input
function Ki = fcn(Ki_ref, y)

Ki = Ki_ref*y;

== matlab function new_model_like_me/Control/Current Control/Old Autotune/PI(z)id/MATLAB Function2 ==
  data: Kaw_ref input; Kaw output; y input
function Kaw = fcn(Kaw_ref, y)

Kaw = Kaw_ref*y;

== matlab function new_model_like_me/Control/Current Control/Old Autotune/PI(z)iq/MATLAB Function1 ==
  data: Ki_ref input; Ki output; y input
function Ki = fcn(Ki_ref, y)

Ki = Ki_ref*y;

== matlab function new_model_like_me/Control/Current Control/Old Autotune/PI(z)iq/MATLAB Function2 ==
  data: Kaw_ref input; Kaw output; y input
function Kaw = fcn(Kaw_ref, y)

Kaw = Kaw_ref*y;

== matlab function new_model_like_me/Control/Speed Control/PI(z)1/MATLAB Function ==
  data: Kp_ref input; Kp output; y input
function Kp = fcn(Kp_ref, y)

Kp = Kp_ref*y;

== matlab function new_model_like_me/Control/Speed Control/PI(z)1/MATLAB Function1 ==
  data: Ki_ref input; Ki output; y input
function Ki = fcn(Ki_ref, y)

Ki = Ki_ref*y;

== matlab function new_model_like_me/Control/Speed Control/PI(z)1/MATLAB Function2 ==
  data: Kaw_ref input; Kaw output; y input
function Kaw = fcn(Kaw_ref, y)

Kaw = Kaw_ref*y;

== matlab function new_model_like_me/Control/Speed Control/Subsystem1/MATLAB Function ==
  data: Kp_omega input; num_omega output; Ki_omega input; Tso input
function num_omega = fcn(Kp_omega, Ki_omega, Tso)

num_omega = (Tso*Ki_omega)/Kp_omega;

== matlab function new_model_like_me/Control/Speed Control/Subsystem1/MATLAB Function1 ==
  data: Kp_omega input; den_omega output; Ki_omega input; Tso input
function den_omega = fcn(Kp_omega, Ki_omega, Tso)

den_omega = [1, ((Tso - Kp_omega/Ki_omega)/(Kp_omega/Ki_omega))];

== stateflow chart new_model_like_me/Control/Task Scheduler ==
  (default) -> (junction 23) : CLK_50us
  (junction 23) -> (junction 17)
  (junction 17) -> (junction 22) [order 2]
  (junction 17) -> (junction 22) [order 1] : [cnt%%2==0]{Task_100us_1;}
  (junction 22) -> (junction 18) [order 2]
  (junction 22) -> (junction 18) [order 1] : [cnt%%2==0]{Task_100us_2;}
  (junction 18) -> (junction 44) [order 1] : [cnt%%20==0]{Task_1ms_1;}
  (junction 18) -> (junction 44) [order 2]
  (junction 44) -> (junction 21) [order 1] : [cnt%%20==0]{Task_1ms_2;}
  (junction 44) -> (junction 21) [order 2]
  (junction 21) -> (junction 34) [order 2]
  (junction 21) -> (junction 16) [order 1] : [1]{cnt++;}
  data: cnt local int32
  events: Task_100us_1 output FUNCTION_CALL_EVENT; Task_100us_2 output FUNCTION_CALL_EVENT; Task_1ms_1 output FUNCTION_CALL_EVENT; CLK_50us input FUNCTION_CALL_EVENT; Task_1ms_2 output FUNCTION_CALL_EVENT

== matlab function new_model_like_me/Control/Current Control/Old Autotune/PI(z)iq/MATLAB Function ==
  data: Kp_ref input; Kp output; y input
function Kp = fcn(Kp_ref, y)

Kp = Kp_ref*y;

== matlab function new_model_like_me/Control/Current Control/Old Autotune/zero_id/MATLAB Function ==
  data: Kp_id input; num_id output; Ki_id input; Tsi input
function num_id = fcn(Kp_id, Ki_id, Tsi)

num_id = (Tsi*Ki_id)/(Kp_id);

== matlab function new_model_like_me/Control/Current Control/Old Autotune/zero_iq/MATLAB Function1 ==
  data: Kp_iq input; num_iq output; Ki_iq input; Tsi input
function num_iq = fcn(Kp_iq, Ki_iq, Tsi)

num_iq = (Tsi*Ki_iq)/(Kp_iq);
